simulink model "Task5"  (R2021a)
settings: Solver=VariableStepAuto  StartTime=0.0  StopTime=10.0  RelTol=1e-3
libraries: fuzblock x1
settings Model: Creator=ejbejaranos  LastModifiedBy=ejbejaranos

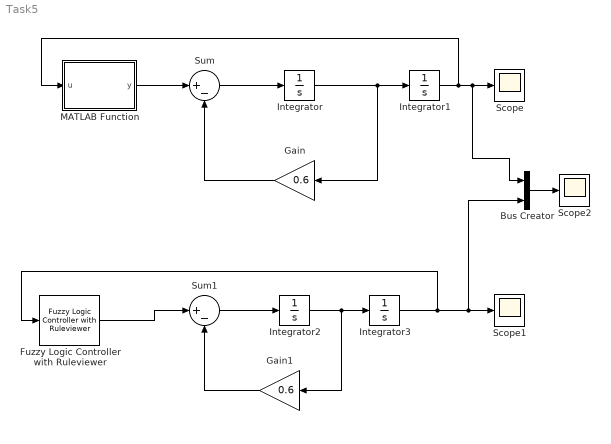
== system Task5 ==
  Bus Creator : BusCreator  Inputs=2
  Fuzzy Logic Controller with Ruleviewer : fuzblock/Fuzzy Logic  Controller  with Ruleviewer  fismatrix=fismat1  Ts=2
  Gain : Gain  Gain=0.6  RndMeth=Convergent
  Gain1 : Gain  Gain=0.6  RndMeth=Convergent
  Integrator : Integrator  InitialCondition=0.5
  Integrator1 : Integrator  InitialCondition=-0.2
  Integrator2 : Integrator  InitialCondition=0.5
  Integrator3 : Integrator  InitialCondition=-0.2
  MATLAB Function : MATLAB Function  TreatAsAtomicUnit=on
  Scope : Scope
  Scope1 : Scope
  Scope2 : Scope
  Sum : Sum  Inputs=|+-
  Sum1 : Sum  Inputs=|+-
  wires:
  Sum/1 -> Integrator/1
  Integrator1/1 -> MATLAB Function/1(u), Bus Creator/1, Scope/1
  Integrator3/1 -> Fuzzy Logic Controller with Ruleviewer/1, Bus Creator/2, Scope1/1
  Bus Creator/1 -> Scope2/1
  Fuzzy Logic Controller with Ruleviewer/1 -> Sum1/1
  Sum1/1 -> Integrator2/1
  Integrator2/1 -> Gain1/1, Integrator3/1
  Gain/1 -> Sum/2
  Integrator/1 -> Gain/1, Integrator1/1
  Gain1/1 -> Sum1/2
  MATLAB Function/1(y) -> Sum/1

== matlab function Task5/MATLAB Function ==
  data: u input; y output
function y = fcn(u)
y=-2*u - u^2;
